simulink model "test1"  (R2018a)
settings: Solver=FixedStepAuto  StartTime=0.0  StopTime=100  FixedStep=step_size  RelTol=1e-3  EnableMultiTasking=on
values from neighbouring files (symbols this model uses):
  alpha1 = 0.995    [DPEFOD.m]
  alpha2 = 0.075    [DPEFOD.m]
  B_bar = [A_hat'*inv(C_hat)*b1_hat;A_hat'*inv(C_hat)*b2_hat;A_hat'*inv(C_hat)*b3_hat;A_hat'*inv(C_hat)*b4_hat]    [DPEFOD.m]
  K_bar = kron(eye(4),A_hat'*inv(C_hat)*A_hat+rho*eye(5))+L_bar    [DPEFOD.m]
  L_bar = kron(L,eye(5))    [DPEFOD.m]
  lambda_0 = zeros(20,1)    [DPEFOD.m]
  theta_0 = zeros(20,1)    [DPEFOD.m]
(part 3 of 5)

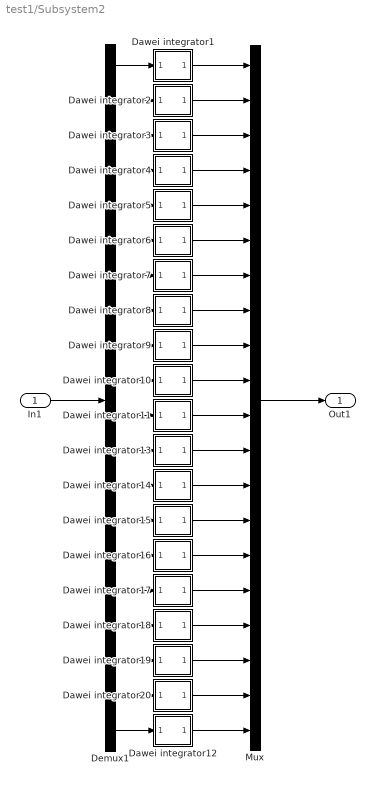
== system test1/Subsystem2 ==
  In1 : Inport
  Dawei integrator1 : Subsystem  mask(Subsystem){alpha=alpha1, gamma=10, wl=1e-3, wh=1e3, k=20, x0=0}
      mask prompts: alpha "Fractional integrator order"; gamma "Edge frequency coefficient"; wl "Frequency lower bound"; wh "Frequency higher bound"; k "Degree of approximation model"; x0 "Initial condition"
      mask help: Fractional-order differentiation with Dawei's hybrid filter.
      mask init: same as test1/Subsystem/Dawei integrator1
      mask Display:
      | %第一种
      | % str='1 \n';
      | % str=[str, '——\n\n\n' ];
      | % disp(str)
      | % str=['s^{', num2str(alpha),'}' ];
      | % disp(str,'texmode','on')
      | %第二种
      | disp(str)
  Dawei integrator10 : Subsystem  mask(Subsystem){alpha=alpha1, gamma=10, wl=1e-3, wh=1e3, k=20, x0=0}
      mask prompts: alpha "Fractional integrator order"; gamma "Edge frequency coefficient"; wl "Frequency lower bound"; wh "Frequency higher bound"; k "Degree of approximation model"; x0 "Initial condition"
      mask help: Fractional-order differentiation with Dawei's hybrid filter.
      mask init: same as test1/Subsystem/Dawei integrator1
      mask Display:
      | %第一种
      | % str='1 \n';
      | % str=[str, '——\n\n\n' ];
      | % disp(str)
      | % str=['s^{', num2str(alpha),'}' ];
      | % disp(str,'texmode','on')
      | %第二种
      | disp(str)
  Dawei integrator11 : Subsystem  mask(Subsystem){alpha=alpha1, gamma=10, wl=1e-3, wh=1e3, k=20, x0=0}
      mask prompts: alpha "Fractional integrator order"; gamma "Edge frequency coefficient"; wl "Frequency lower bound"; wh "Frequency higher bound"; k "Degree of approximation model"; x0 "Initial condition"
      mask help: Fractional-order differentiation with Dawei's hybrid filter.
      mask init: same as test1/Subsystem/Dawei integrator1
      mask Display:
      | %第一种
      | % str='1 \n';
      | % str=[str, '——\n\n\n' ];
      | % disp(str)
      | % str=['s^{', num2str(alpha),'}' ];
      | % disp(str,'texmode','on')
      | %第二种
      | disp(str)
  Dawei integrator12 : Subsystem  mask(Subsystem){alpha=alpha1, gamma=10, wl=1e-3, wh=1e3, k=20, x0=0}
      mask prompts: alpha "Fractional integrator order"; gamma "Edge frequency coefficient"; wl "Frequency lower bound"; wh "Frequency higher bound"; k "Degree of approximation model"; x0 "Initial condition"
      mask help: Fractional-order differentiation with Dawei's hybrid filter.
      mask init: same as test1/Subsystem/Dawei integrator1
      mask Display:
      | %第一种
      | % str='1 \n';
      | % str=[str, '——\n\n\n' ];
      | % disp(str)
      | % str=['s^{', num2str(alpha),'}' ];
      | % disp(str,'texmode','on')
      | %第二种
      | disp(str)
  Dawei integrator13 : Subsystem  mask(Subsystem){alpha=alpha1, gamma=10, wl=1e-3, wh=1e3, k=20, x0=0}
      mask prompts: alpha "Fractional integrator order"; gamma "Edge frequency coefficient"; wl "Frequency lower bound"; wh "Frequency higher bound"; k "Degree of approximation model"; x0 "Initial condition"
      mask help: Fractional-order differentiation with Dawei's hybrid filter.
      mask init: same as test1/Subsystem/Dawei integrator1
      mask Display:
      | %第一种
      | % str='1 \n';
      | % str=[str, '——\n\n\n' ];
      | % disp(str)
      | % str=['s^{', num2str(alpha),'}' ];
      | % disp(str,'texmode','on')
      | %第二种
      | disp(str)
  Dawei integrator14 : Subsystem  mask(Subsystem){alpha=alpha1, gamma=10, wl=1e-3, wh=1e3, k=20, x0=0}
      mask prompts: alpha "Fractional integrator order"; gamma "Edge frequency coefficient"; wl "Frequency lower bound"; wh "Frequency higher bound"; k "Degree of approximation model"; x0 "Initial condition"
      mask help: Fractional-order differentiation with Dawei's hybrid filter.
      mask init: same as test1/Subsystem/Dawei integrator1
      mask Display:
      | %第一种
      | % str='1 \n';
      | % str=[str, '——\n\n\n' ];
      | % disp(str)
      | % str=['s^{', num2str(alpha),'}' ];
      | % disp(str,'texmode','on')
      | %第二种
      | disp(str)
  Dawei integrator15 : Subsystem  mask(Subsystem){alpha=alpha1, gamma=10, wl=1e-3, wh=1e3, k=20, x0=0}
      mask prompts: alpha "Fractional integrator order"; gamma "Edge frequency coefficient"; wl "Frequency lower bound"; wh "Frequency higher bound"; k "Degree of approximation model"; x0 "Initial condition"
      mask help: Fractional-order differentiation with Dawei's hybrid filter.
      mask init: same as test1/Subsystem/Dawei integrator1
      mask Display:
      | %第一种
      | % str='1 \n';
      | % str=[str, '——\n\n\n' ];
      | % disp(str)
      | % str=['s^{', num2str(alpha),'}' ];
      | % disp(str,'texmode','on')
      | %第二种
      | disp(str)
  Dawei integrator16 : Subsystem  mask(Subsystem){alpha=alpha1, gamma=10, wl=1e-3, wh=1e3, k=20, x0=0}
      mask prompts: alpha "Fractional integrator order"; gamma "Edge frequency coefficient"; wl "Frequency lower bound"; wh "Frequency higher bound"; k "Degree of approximation model"; x0 "Initial condition"
      mask help: Fractional-order differentiation with Dawei's hybrid filter.
      mask init: same as test1/Subsystem/Dawei integrator1
      mask Display:
      | %第一种
      | % str='1 \n';
      | % str=[str, '——\n\n\n' ];
      | % disp(str)
      | % str=['s^{', num2str(alpha),'}' ];
      | % disp(str,'texmode','on')
      | %第二种
      | disp(str)
  Dawei integrator17 : Subsystem  mask(Subsystem){alpha=alpha1, gamma=10, wl=1e-3, wh=1e3, k=20, x0=0}
      mask prompts: alpha "Fractional integrator order"; gamma "Edge frequency coefficient"; wl "Frequency lower bound"; wh "Frequency higher bound"; k "Degree of approximation model"; x0 "Initial condition"
      mask help: Fractional-order differentiation with Dawei's hybrid filter.
      mask init: same as test1/Subsystem/Dawei integrator1
      mask Display:
      | %第一种
      | % str='1 \n';
      | % str=[str, '——\n\n\n' ];
      | % disp(str)
      | % str=['s^{', num2str(alpha),'}' ];
      | % disp(str,'texmode','on')
      | %第二种
      | disp(str)
  Dawei integrator18 : Subsystem  mask(Subsystem){alpha=alpha1, gamma=10, wl=1e-3, wh=1e3, k=20, x0=0}
      mask prompts: alpha "Fractional integrator order"; gamma "Edge frequency coefficient"; wl "Frequency lower bound"; wh "Frequency higher bound"; k "Degree of approximation model"; x0 "Initial condition"
      mask help: Fractional-order differentiation with Dawei's hybrid filter.
      mask init: same as test1/Subsystem/Dawei integrator1
      mask Display:
      | %第一种
      | % str='1 \n';
      | % str=[str, '——\n\n\n' ];
      | % disp(str)
      | % str=['s^{', num2str(alpha),'}' ];
      | % disp(str,'texmode','on')
      | %第二种
      | disp(str)
  Dawei integrator19 : Subsystem  mask(Subsystem){alpha=alpha1, gamma=10, wl=1e-3, wh=1e3, k=20, x0=0}
      mask prompts: alpha "Fractional integrator order"; gamma "Edge frequency coefficient"; wl "Frequency lower bound"; wh "Frequency higher bound"; k "Degree of approximation model"; x0 "Initial condition"
      mask help: Fractional-order differentiation with Dawei's hybrid filter.
      mask init: same as test1/Subsystem/Dawei integrator1
      mask Display:
      | %第一种
      | % str='1 \n';
      | % str=[str, '——\n\n\n' ];
      | % disp(str)
      | % str=['s^{', num2str(alpha),'}' ];
      | % disp(str,'texmode','on')
      | %第二种
      | disp(str)
  Dawei integrator2 : Subsystem  mask(Subsystem){alpha=alpha1, gamma=10, wl=1e-3, wh=1e3, k=20, x0=0}
      mask prompts: alpha "Fractional integrator order"; gamma "Edge frequency coefficient"; wl "Frequency lower bound"; wh "Frequency higher bound"; k "Degree of approximation model"; x0 "Initial condition"
      mask help: Fractional-order differentiation with Dawei's hybrid filter.
      mask init: same as test1/Subsystem/Dawei integrator1
      mask Display:
      | %第一种
      | % str='1 \n';
      | % str=[str, '——\n\n\n' ];
      | % disp(str)
      | % str=['s^{', num2str(alpha),'}' ];
      | % disp(str,'texmode','on')
      | %第二种
      | disp(str)
  Dawei integrator20 : Subsystem  mask(Subsystem){alpha=alpha1, gamma=10, wl=1e-3, wh=1e3, k=20, x0=0}
      mask prompts: alpha "Fractional integrator order"; gamma "Edge frequency coefficient"; wl "Frequency lower bound"; wh "Frequency higher bound"; k "Degree of approximation model"; x0 "Initial condition"
      mask help: Fractional-order differentiation with Dawei's hybrid filter.
      mask init: same as test1/Subsystem/Dawei integrator1
      mask Display:
      | %第一种
      | % str='1 \n';
      | % str=[str, '——\n\n\n' ];
      | % disp(str)
      | % str=['s^{', num2str(alpha),'}' ];
      | % disp(str,'texmode','on')
      | %第二种
      | disp(str)
  Dawei integrator3 : Subsystem  mask(Subsystem){alpha=alpha1, gamma=10, wl=1e-3, wh=1e3, k=20, x0=0}
      mask prompts: alpha "Fractional integrator order"; gamma "Edge frequency coefficient"; wl "Frequency lower bound"; wh "Frequency higher bound"; k "Degree of approximation model"; x0 "Initial condition"
      mask help: Fractional-order differentiation with Dawei's hybrid filter.
      mask init: same as test1/Subsystem/Dawei integrator1
      mask Display:
      | %第一种
      | % str='1 \n';
      | % str=[str, '——\n\n\n' ];
      | % disp(str)
      | % str=['s^{', num2str(alpha),'}' ];
      | % disp(str,'texmode','on')
      | %第二种
      | disp(str)
  Dawei integrator4 : Subsystem  mask(Subsystem){alpha=alpha1, gamma=10, wl=1e-3, wh=1e3, k=20, x0=0}
      mask prompts: alpha "Fractional integrator order"; gamma "Edge frequency coefficient"; wl "Frequency lower bound"; wh "Frequency higher bound"; k "Degree of approximation model"; x0 "Initial condition"
      mask help: Fractional-order differentiation with Dawei's hybrid filter.
      mask init: same as test1/Subsystem/Dawei integrator1
      mask Display:
      | %第一种
      | % str='1 \n';
      | % str=[str, '——\n\n\n' ];
      | % disp(str)
      | % str=['s^{', num2str(alpha),'}' ];
      | % disp(str,'texmode','on')
      | %第二种
      | disp(str)
  Dawei integrator5 : Subsystem  mask(Subsystem){alpha=alpha1, gamma=10, wl=1e-3, wh=1e3, k=20, x0=0}
      mask prompts: alpha "Fractional integrator order"; gamma "Edge frequency coefficient"; wl "Frequency lower bound"; wh "Frequency higher bound"; k "Degree of approximation model"; x0 "Initial condition"
      mask help: Fractional-order differentiation with Dawei's hybrid filter.
      mask init: same as test1/Subsystem/Dawei integrator1
      mask Display:
      | %第一种
      | % str='1 \n';
      | % str=[str, '——\n\n\n' ];
      | % disp(str)
      | % str=['s^{', num2str(alpha),'}' ];
      | % disp(str,'texmode','on')
      | %第二种
      | disp(str)
  Dawei integrator6 : Subsystem  mask(Subsystem){alpha=alpha1, gamma=10, wl=1e-3, wh=1e3, k=20, x0=0}
      mask prompts: alpha "Fractional integrator order"; gamma "Edge frequency coefficient"; wl "Frequency lower bound"; wh "Frequency higher bound"; k "Degree of approximation model"; x0 "Initial condition"
      mask help: Fractional-order differentiation with Dawei's hybrid filter.
      mask init: same as test1/Subsystem/Dawei integrator1
      mask Display:
      | %第一种
      | % str='1 \n';
      | % str=[str, '——\n\n\n' ];
      | % disp(str)
      | % str=['s^{', num2str(alpha),'}' ];
      | % disp(str,'texmode','on')
      | %第二种
      | disp(str)
  Dawei integrator7 : Subsystem  mask(Subsystem){alpha=alpha1, gamma=10, wl=1e-3, wh=1e3, k=20, x0=0}
      mask prompts: alpha "Fractional integrator order"; gamma "Edge frequency coefficient"; wl "Frequency lower bound"; wh "Frequency higher bound"; k "Degree of approximation model"; x0 "Initial condition"
      mask help: Fractional-order differentiation with Dawei's hybrid filter.
      mask init: same as test1/Subsystem/Dawei integrator1
      mask Display:
      | %第一种
      | % str='1 \n';
      | % str=[str, '——\n\n\n' ];
      | % disp(str)
      | % str=['s^{', num2str(alpha),'}' ];
      | % disp(str,'texmode','on')
      | %第二种
      | disp(str)
  Dawei integrator8 : Subsystem  mask(Subsystem){alpha=alpha1, gamma=10, wl=1e-3, wh=1e3, k=20, x0=0}
      mask prompts: alpha "Fractional integrator order"; gamma "Edge frequency coefficient"; wl "Frequency lower bound"; wh "Frequency higher bound"; k "Degree of approximation model"; x0 "Initial condition"
      mask help: Fractional-order differentiation with Dawei's hybrid filter.
      mask init: same as test1/Subsystem/Dawei integrator1
      mask Display:
      | %第一种
      | % str='1 \n';
      | % str=[str, '——\n\n\n' ];
      | % disp(str)
      | % str=['s^{', num2str(alpha),'}' ];
      | % disp(str,'texmode','on')
      | %第二种
      | disp(str)
  Dawei integrator9 : Subsystem  mask(Subsystem){alpha=alpha1, gamma=10, wl=1e-3, wh=1e3, k=20, x0=0}
      mask prompts: alpha "Fractional integrator order"; gamma "Edge frequency coefficient"; wl "Frequency lower bound"; wh "Frequency higher bound"; k "Degree of approximation model"; x0 "Initial condition"
      mask help: Fractional-order differentiation with Dawei's hybrid filter.
      mask init: same as test1/Subsystem/Dawei integrator1
      mask Display:
      | %第一种
      | % str='1 \n';
      | % str=[str, '——\n\n\n' ];
      | % disp(str)
      | % str=['s^{', num2str(alpha),'}' ];
      | % disp(str,'texmode','on')
      | %第二种
      | disp(str)
  Demux1 : Demux  Outputs=20
  Mux : Mux  Inputs=20
  Out1 : Outport
  wires:
  Demux1/4 -> Dawei integrator4/1(In1)
  Demux1/16 -> Dawei integrator17/1(In1)
  Dawei integrator13/1(Out1) -> Mux/12
  Demux1/15 -> Dawei integrator16/1(In1)
  Dawei integrator12/1(Out1) -> Mux/20
  Dawei integrator15/1(Out1) -> Mux/14
  Mux/1 -> Out1/1
  Dawei integrator8/1(Out1) -> Mux/8
  Demux1/19 -> Dawei integrator20/1(In1)
  Dawei integrator11/1(Out1) -> Mux/11
  Dawei integrator3/1(Out1) -> Mux/3
  Dawei integrator5/1(Out1) -> Mux/5
  Dawei integrator19/1(Out1) -> Mux/18
  Dawei integrator6/1(Out1) -> Mux/6
  Dawei integrator2/1(Out1) -> Mux/2
  Demux1/11 -> Dawei integrator11/1(In1)
  Dawei integrator7/1(Out1) -> Mux/7
  Demux1/18 -> Dawei integrator19/1(In1)
  Demux1/12 -> Dawei integrator13/1(In1)
  Demux1/3 -> Dawei integrator3/1(In1)
  Demux1/7 -> Dawei integrator7/1(In1)
  Dawei integrator17/1(Out1) -> Mux/16
  Dawei integrator18/1(Out1) -> Mux/17
  Dawei integrator14/1(Out1) -> Mux/13
  Dawei integrator10/1(Out1) -> Mux/10
  Dawei integrator20/1(Out1) -> Mux/19
  Dawei integrator9/1(Out1) -> Mux/9
  Demux1/10 -> Dawei integrator10/1(In1)
  Dawei integrator1/1(Out1) -> Mux/1
  Demux1/8 -> Dawei integrator8/1(In1)
  Demux1/14 -> Dawei integrator15/1(In1)
  Dawei integrator16/1(Out1) -> Mux/15
  Demux1/17 -> Dawei integrator18/1(In1)
  Demux1/9 -> Dawei integrator9/1(In1)
  Demux1/20 -> Dawei integrator12/1(In1)
  In1/1 -> Demux1/1
  Dawei integrator4/1(Out1) -> Mux/4
  Demux1/2 -> Dawei integrator2/1(In1)
  Demux1/5 -> Dawei integrator5/1(In1)
  Demux1/13 -> Dawei integrator14/1(In1)
  Demux1/1 -> Dawei integrator1/1(In1)
  Demux1/6 -> Dawei integrator6/1(In1)
